simulink model "pd_sim"  (R2022a)
settings: Solver=VariableStepAuto  StartTime=0.0  StopTime=1.0  RelTol=1e-3
undefined symbols (not defined in the file): a1, a2, B, dq0, dtheta0, K, Kp, Ks, Kt, Kv, m1, m2, q0, r_d, S, theta0
settings Model: Creator=mathe  LastModifiedBy=mathe

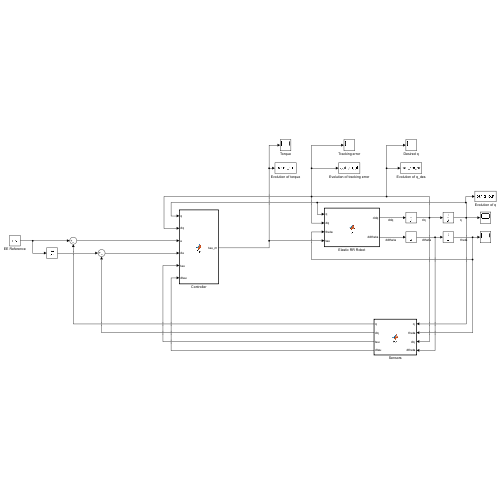
[thumbnail: Simulink's stored preview of the top-level diagram]
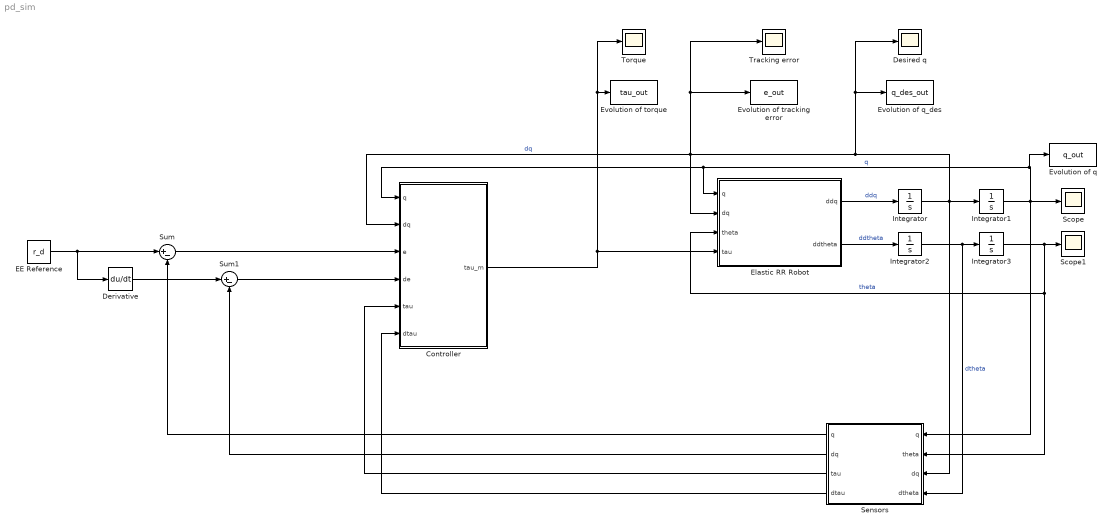
== system pd_sim ==
  Controller : MATLAB Function  TreatAsAtomicUnit=on
  Derivative : Derivative
  Desired q : Scope
  EE Reference : Constant  Value=r_d
  Elastic RR Robot : MATLAB Function  TreatAsAtomicUnit=on
  Evolution of q : ToWorkspace  VariableName=q_out  SaveFormat=Timeseries  SampleTime=-1
  Evolution of q_des : ToWorkspace  VariableName=q_des_out  SaveFormat=Timeseries  SampleTime=-1
  Evolution of torque : ToWorkspace  VariableName=tau_out  SaveFormat=Timeseries  SampleTime=-1
  Evolution of tracking error : ToWorkspace  VariableName=e_out  SaveFormat=Timeseries  SampleTime=-1
  Integrator : Integrator  InitialCondition=dq0
  Integrator1 : Integrator  InitialCondition=q0
  Integrator2 : Integrator  InitialCondition=dtheta0
  Integrator3 : Integrator  InitialCondition=theta0
  Scope : Scope
  Scope1 : Scope
  Sensors : MATLAB Function  TreatAsAtomicUnit=on
  Sum : Sum  Inputs=|+-
  Sum1 : Sum  Inputs=|+-
  Torque : Scope
  Tracking error : Scope
  wires:
  Elastic RR Robot/1(ddq) -> Integrator/1  "ddq"
  Integrator/1 -> Elastic RR Robot/2(dq), Controller/2(dq), Tracking error/1, Evolution of tracking error/1, Evolution of q_des/1, Desired q/1, Sensors/3("dq "), Integrator1/1  "dq"
  Integrator2/1 -> Sensors/4(dtheta), Integrator3/1  "dtheta"
  Elastic RR Robot/2(ddtheta) -> Integrator2/1  "ddtheta"
  Integrator3/1 -> Scope1/1, Sensors/2(theta), Elastic RR Robot/3(theta)  "theta"
  Integrator1/1 -> Sensors/1("q "), Scope/1, Elastic RR Robot/1(q), Controller/1(q), Evolution of q/1  "q"
  Controller/1(tau_m) -> Torque/1, Evolution of torque/1, Elastic RR Robot/4(tau)
  EE Reference/1 -> Derivative/1, Sum/1
  Derivative/1 -> Sum1/1
  Sum/1 -> Controller/3(e)
  Sum1/1 -> Controller/4(de)
  Sensors/3(tau) -> Controller/5(tau)
  Sensors/4(dtau) -> Controller/6(dtau)
  Sensors/1(q) -> Sum/2
  Sensors/2(dq) -> Sum1/2

== matlab function pd_sim/Controller ==
  data: q input; dq input; e input; tau_m output; de input; tau input; dtau input; K parameter; B parameter; S parameter; m1 parameter; m2 parameter; a1 parameter; a2 parameter; Kp parameter; Kv parameter; Ks parameter; Kt parameter
function tau_m = fcn(q, dq, e, de, tau, dtau, K, B, S, m1, m2, a1, a2, ...
    Kp, Kv, Ks, Kt)

% Compute dynamic matrices
[M, C, G] = dynamics(q, dq, m1, m2, a1, a2);

% PD Control
tau_d = Kp*e + Kv*de;

% Torque Control
tau_m = tau_d + Kt*(tau_d - tau) + Ks*dtau;

== matlab function pd_sim/Elastic RR Robot ==
  data: q input; ddq output; dq input; theta input; tau input; ddtheta output; K parameter; B parameter; S parameter; m1 parameter; m2 parameter; a1 parameter; a2 parameter
function [ddq, ddtheta] = fcn(q, dq, theta, tau, K, B, S, m1, m2, a1, a2)

% Compute dynamic matrices
[M, C, G] = dynamics(q, dq, m1, m2, a1, a2);

% State evolutions
ddq = M\(S.'*K*(theta - q) - C*dq - G);
ddtheta = B\(tau - K*(theta - q));

== matlab function pd_sim/Sensors ==
  data: q input; theta input; dq input; dtheta input; q output; dq output; tau output; K parameter; dtau output
function [q, dq, tau, dtau] = fcn(q, theta, dq, dtheta, K)

tau = K*(theta - q);
dtau = K*(dtheta - dq);
